simulink model "pid_iir_demo"  (R2018a)
settings: Solver=ode23tb  StartTime=0.0  StopTime=10  MaxStep=1e-4  RelTol=1e-3
undefined symbols (not defined in the file): D, I, N, P, T
libraries: simulink x2
settings Model: Creator=joe  LastModifiedBy=joe

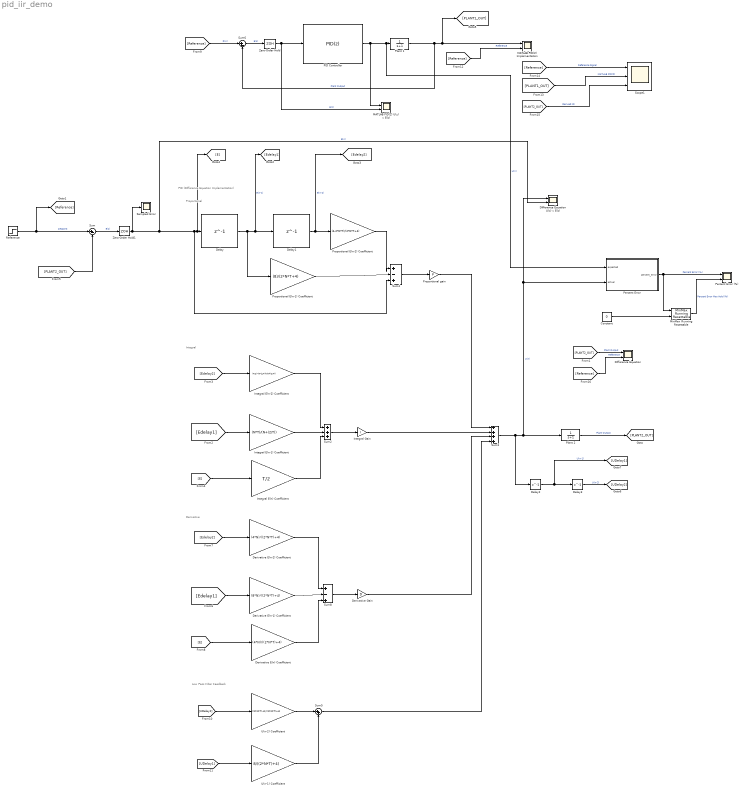
== system pid_iir_demo ==
  note: PID (Difference Equation Implementation)
  note: Low Pass Filter Feedback
  note: Integral
  note: Proportional
  note: Derivative
  Constant : Constant  Value=0
  Delay{,1..3} (4 alike) : Delay  DelayLength=1
  Derivative E(n) Coefficient : Gain  Gain=(4*N)/((2*N*T)+4)
  Derivative E(n-1) Coefficient : Gain  Gain=(8*N)/((2*N*T)+4)
  Derivative E(n-2) Coefficient : Gain  Gain=(4*N)/((2*N*T)+4)
  Derivative Gain : Gain  Gain=D
  Difference Equation : Scope  NumInputPorts=2
  Difference Equation U(z) v E(z) : Scope  NumInputPorts=2
  Integral E(n) Coefficient : Gain  Gain=T/2
  Integral E(n-1) Coefficient : Gain  Gain=(N*T)/(N+(2/T))
  Integral E(n-2) Coefficient : Gain  Gain=(T/2)*(N-(2/T))/(N+(2/T))
  Integral Gain : Gain  Gain=I
  MATLAB PID(Z) Implementation : Scope  NumInputPorts=2
  MATLAB PID(Z) U(z) v E(z) : Scope  NumInputPorts=2
  MinMax Running Resettable : simulink/Math Operations/MinMax Running Resettable  Function=max  vinit=0.0
  PID Controller : simulink/Continuous/PID Controller  Controller=PID  TimeDomain=Discrete-time  SampleTime=-1  IntegratorMethod=Trapezoidal  FilterMethod=Trapezoidal  Form=Parallel  UseFilter=on  ControllerParametersSource=internal  P=P  I=I  D=D  N=N  InitialConditionSource=internal  InitialConditionForIntegrator=0  InitialConditionForFilter=0  ExternalReset=none  LimitOutput=off  UpperSaturationLimit=inf  LowerSaturationLimit=-inf  LinearizeAsGain=on  AntiWindupMode=none  Kb=1  TrackingMode=off  Kt=1  PParamMin=[]  PParamMax=[]  IParamMin=[]  IParamMax=[]  DParamMin=[]  DParamMax=[]  NParamMin=[]  NParamMax=[]  KbParamMin=[]  KbParamMax=[]  KtParamMin=[]  KtParamMax=[]  POutMin=[]  POutMax=[]  IOutMin=[]  IOutMax=[]  DOutMin=[]  DOutMax=[]  NOutMin=[]  NOutMax=[]  KbOutMin=[]  KbOutMax=[]  KtOutMin=[]  KtOutMax=[]  IntegratorOutMin=[]  IntegratorOutMax=[]  FilterOutMin=[]  FilterOutMax=[]  SumOutMin=[]  SumOutMax=[]  SumI1OutMin=[]  SumI1OutMax=[]  SumI2OutMin=[]  SumI2OutMax=[]  SumI3OutMin=[]  SumI3OutMax=[]  SumDOutMin=[]  SumDOutMax=[]  SaturationOutMin=[]  SaturationOutMax=[]  IntegratorContinuousStateAttributes=''  IntegratorStateMustResolveToSignalObject=off  IntegratorRTWStateStorageClass=Auto  FilterContinuousStateAttributes=''  FilterStateMustResolveToSignalObject=off  FilterRTWStateStorageClass=Auto  DifferentiatorICPrevScaledInput=0  DifferentiatorOutMin=[]  DifferentiatorOutMax=[]  FilterDiffOutCoefMin=[]  FilterDiffOutCoefMax=[]  SumDenOutMin=[]  SumDenOutMax=[]  SumNumOutMin=[]  SumNumOutMax=[]  ReciprocalOutMin=[]  ReciprocalOutMax=[]  DivideOutMin=[]  DivideOutMax=[]  TunerSelectOption=Transfer Function Based (PID Tuner App)
  Percent Error : MATLAB Function  TreatAsAtomicUnit=on
  Percent Error (%) : Scope  NumInputPorts=2
  Plant 1 : TransferFcn  Denominator=[1 1]
  Plant 2 : TransferFcn  Denominator=[1 1]
  Proportional E(n-1) Coefficient : Gain  Gain=(8)/(2*N*T+4)
  Proportional E(n-2) Coefficient : Gain  Gain=(4-2*N*T)/(2*N*T+4)
  Proportional gain : Gain  Gain=P
  Reference : Step  SampleTime=0
  Sampled Error : Scope
  Scope1 : Scope  NumInputPorts=3
  Sum : Sum  Inputs=|+-
  Sum2 : Sum  Inputs=3
  Sum3 : Sum  Inputs=4
  Sum4 : Sum  Inputs=|+-+
  Sum5 : Sum  Inputs=|++
  Sum6 : Sum  Inputs=|+-
  Sum8 : Sum  Inputs=|+-+
  U(n-1) Coefficient : Gain  Gain=8/((2*N*T)+4)
  U(n-2) Coefficient : Gain  Gain=((2*N*T)-4)/((2*N*T)+4)
  Zero-Order Hold : ZeroOrderHold  SampleTime=T
  Zero-Order Hold1 : ZeroOrderHold  SampleTime=T
  wires:
  Sum/1 -> Zero-Order Hold1/1  "E(s)"
  Delay/1 -> Delay1/1, [Edelay1], Proportional E(n-1) Coefficient/1  "E(n-1)"
  Delay1/1 -> Proportional E(n-2) Coefficient/1, [Edelay2]  "E(n-2)"
  Proportional E(n-2) Coefficient/1 -> Sum4/1
  Proportional E(n-1) Coefficient/1 -> Sum4/2
  Sum4/1 -> Proportional gain/1
  Plant 2/1 -> [PLANT2_OUT]  "Plant Output"
  Sum2/1 -> Integral Gain/1
  Integral E(n-1) Coefficient/1 -> Sum2/2
  Integral E(n-2) Coefficient/1 -> Sum2/1
  [Edelay1] -> Integral E(n-1) Coefficient/1
  [Edelay2] -> Integral E(n-2) Coefficient/1
  [E] -> Integral E(n) Coefficient/1
  Integral E(n) Coefficient/1 -> Sum2/3
  [PLANT2_OUT] -> Sum/2
  Proportional gain/1 -> Sum3/1
  Integral Gain/1 -> Sum3/2
  Sum3/1 -> Difference Equation U(z) v E(z)/1, Percent Error/2(actual), Plant 2/1, Delay2/1  "U(n)"
  [E] -> Derivative E(n) Coefficient/1
  Derivative Gain/1 -> Sum3/3
  [Edelay1] -> Derivative E(n-1) Coefficient/1
  Derivative E(n-1) Coefficient/1 -> Sum8/2
  [Edelay2] -> Derivative E(n-2) Coefficient/1
  Derivative E(n) Coefficient/1 -> Sum8/3
  Delay2/1 -> [UDelay1], Delay3/1  "U(n-1)"
  Delay3/1 -> [UDelay2]  "U(n-2)"
  [UDelay1] -> U(n-1) Coefficient/1
  [UDelay2] -> U(n-2) Coefficient/1
  U(n-2) Coefficient/1 -> Sum5/1
  U(n-1) Coefficient/1 -> Sum5/2
  Sum5/1 -> Sum3/4
  Sum6/1 -> Zero-Order Hold/1  "E(s)"
  Plant 1/1 -> [PLANT1_OUT], MATLAB PID(Z) Implementation/1, Sum6/2  "Plant Output"
  [Reference] -> Sum6/1  "R(s)"
  [Reference] -> MATLAB PID(Z) Implementation/2  "Reference"
  [Reference] -> Scope1/1  "Reference Signal"
  [PLANT1_OUT] -> Scope1/2  "MATLAB PID(Z)"
  [PLANT2_OUT] -> Scope1/3  "Derived IIR"
  PID Controller/1 -> MATLAB PID(Z) U(z) v E(z)/1, Percent Error/1(expected), Plant 1/1  "U(z)"
  Reference/1 -> Sum/1, [Reference]  "setpoint"
  Zero-Order Hold/1 -> MATLAB PID(Z) U(z) v E(z)/2, PID Controller/1  "E(z)"
  Zero-Order Hold1/1 -> Sampled Error/1, Difference Equation U(z) v E(z)/2, Sum4/3, [E], Delay/1  "E(n)"
  Derivative E(n-2) Coefficient/1 -> Sum8/1
  Sum8/1 -> Derivative Gain/1
  [PLANT2_OUT] -> Difference Equation/1  "Plant Output"
  [Reference] -> Difference Equation/2  "Reference"
  Percent Error/1(percent_error) -> MinMax Running Resettable/1, Percent Error (%)/1  "Percent Error (%)"
  MinMax Running Resettable/1 -> Percent Error (%)/2  "Percent Error Max Hold (%)"
  Constant/1 -> MinMax Running Resettable/2

== matlab function pid_iir_demo/Percent Error ==
  data: expected input; percent_error output; actual input
function percent_error = fcn(expected,actual)

percent_error = abs((actual-expected)/expected)*100;
